simulink model "generic_src"  (Simulink 10.3)
settings: Solver=ode45  StartTime=0.0  StopTime=inf  RelTol=1e-3  EnableMultiTasking=on
undefined symbols (not defined in the file or in its folder): Area_Front, Area_Rear, ay_max_off, ay_max_on, ay_per_mu_max_off, ay_per_mu_max_on, Brake_ratio, brake_valve_ctrl_kP, cat1mode1_higher, cat1mode1_lower, cat1mode2_higher, cat1mode2_lower, cat1mode3_higher, cat1mode3_lower, cat2mode1_higher, cat2mode1_lower, cat2mode2_higher, cat2mode2_lower, cat2mode3_higher, cat2mode3_lower, delta_vel, diff_lock_fac, diff_lock_off, diff_lock_on, ESP_ctrl_kD, ESP_ctrl_kI, ESP_ctrl_kP, ESP_ctrl_restore_kI, ESP_min_throttle_fac, f_ax, f_slip, g, higherlimit_highvel, higherlimit_lowvel, highervel_fac, highervelocity_fac, InitialConditionForIntegrator, limit_acc, limit_selectlow, limit_starting, limit_vdiff, locktime_throttle, lowerlimit_highvel, lowerlimit_lowvel, lowervel_fac, lowervelocity_fac, min_throttle, MPS2KMPH, MSR_ctrl_kD, MSR_ctrl_kI, MSR_ctrl_kP, MSR_min_throttle_fac, PID_kP_sideslip, PID_kP_yawrate, RADpS2RpM, rBrake, RpM2RADpS, SH_SL_switch, sideslip_vel_corr, sidesplip_deviation_max ... (+35)
libraries: CarMaker4SL x137, simulink x57, simulink_extras x6
(part 6 of 12)

== system generic_src/CarMaker/IPG Vehicle/PowerTrain/PTControl Example/PTControl_In/CreateBus PTC GearboxIn5 ==
  In : Inport
  BusCreator : BusCreator  Inputs=20
  Demux : Demux  Outputs=20
      settings: DisplayOption=none
  Out : Outport  VectorParamsAs1DForOutWhenUnconnected=off
  wires:
  Demux/20 -> BusCreator/20  "PTC GearboxIn5 Clutch_dis i_TrqIn2Out"
  Demux/19 -> BusCreator/19  "PTC GearboxIn5 Clutch_dis Trq_out"
  Demux/18 -> BusCreator/18  "PTC GearboxIn5 Clutch_dis Trq_in"
  Demux/17 -> BusCreator/17  "PTC GearboxIn5 Clutch_dis rotv_out"
  Demux/16 -> BusCreator/16  "PTC GearboxIn5 Clutch_dis rotv_in"
  Demux/15 -> BusCreator/15  "PTC GearboxIn5 Clutch_dis Pos"
  Demux/14 -> BusCreator/14  "PTC GearboxIn5 Clutch i_TrqIn2Out"
  Demux/13 -> BusCreator/13  "PTC GearboxIn5 Clutch Trq_out"
  Demux/12 -> BusCreator/12  "PTC GearboxIn5 Clutch Trq_in"
  Demux/11 -> BusCreator/11  "PTC GearboxIn5 Clutch rotv_out"
  Demux/10 -> BusCreator/10  "PTC GearboxIn5 Clutch rotv_in"
  Demux/9 -> BusCreator/9  "PTC GearboxIn5 Clutch Pos"
  Demux/8 -> BusCreator/8  "PTC GearboxIn5 Trq_out"
  Demux/7 -> BusCreator/7  "PTC GearboxIn5 Trq_in"
  Demux/6 -> BusCreator/6  "PTC GearboxIn5 rotv_out"
  Demux/5 -> BusCreator/5  "PTC GearboxIn5 rotv_in"
  Demux/4 -> BusCreator/4  "PTC GearboxIn5 i"
  Demux/3 -> BusCreator/3  "PTC GearboxIn5 Trq_DriveSrc_trg"
  Demux/2 -> BusCreator/2  "PTC GearboxIn5 GearNo_dis"
  Demux/1 -> BusCreator/1  "PTC GearboxIn5 GearNo"
  BusCreator/1 -> Out/1
  In/1 -> Demux/1

== system generic_src/CarMaker/IPG Vehicle/PowerTrain/PTControl Example/PTControl_In/CreateBus PTC GearboxIn6 ==
  In : Inport
  BusCreator : BusCreator  Inputs=20
  Demux : Demux  Outputs=20
      settings: DisplayOption=none
  Out : Outport  VectorParamsAs1DForOutWhenUnconnected=off
  wires:
  Demux/20 -> BusCreator/20  "PTC GearboxIn6 Clutch_dis i_TrqIn2Out"
  Demux/19 -> BusCreator/19  "PTC GearboxIn6 Clutch_dis Trq_out"
  Demux/18 -> BusCreator/18  "PTC GearboxIn6 Clutch_dis Trq_in"
  Demux/17 -> BusCreator/17  "PTC GearboxIn6 Clutch_dis rotv_out"
  Demux/16 -> BusCreator/16  "PTC GearboxIn6 Clutch_dis rotv_in"
  Demux/15 -> BusCreator/15  "PTC GearboxIn6 Clutch_dis Pos"
  Demux/14 -> BusCreator/14  "PTC GearboxIn6 Clutch i_TrqIn2Out"
  Demux/13 -> BusCreator/13  "PTC GearboxIn6 Clutch Trq_out"
  Demux/12 -> BusCreator/12  "PTC GearboxIn6 Clutch Trq_in"
  Demux/11 -> BusCreator/11  "PTC GearboxIn6 Clutch rotv_out"
  Demux/10 -> BusCreator/10  "PTC GearboxIn6 Clutch rotv_in"
  Demux/9 -> BusCreator/9  "PTC GearboxIn6 Clutch Pos"
  Demux/8 -> BusCreator/8  "PTC GearboxIn6 Trq_out"
  Demux/7 -> BusCreator/7  "PTC GearboxIn6 Trq_in"
  Demux/6 -> BusCreator/6  "PTC GearboxIn6 rotv_out"
  Demux/5 -> BusCreator/5  "PTC GearboxIn6 rotv_in"
  Demux/4 -> BusCreator/4  "PTC GearboxIn6 i"
  Demux/3 -> BusCreator/3  "PTC GearboxIn6 Trq_DriveSrc_trg"
  Demux/2 -> BusCreator/2  "PTC GearboxIn6 GearNo_dis"
  Demux/1 -> BusCreator/1  "PTC GearboxIn6 GearNo"
  BusCreator/1 -> Out/1
  In/1 -> Demux/1

== system generic_src/CarMaker/IPG Vehicle/PowerTrain/PTControl Example/PTControl_In/CreateBus PTC GearboxIn7 ==
  In : Inport
  BusCreator : BusCreator  Inputs=20
  Demux : Demux  Outputs=20
      settings: DisplayOption=none
  Out : Outport  VectorParamsAs1DForOutWhenUnconnected=off
  wires:
  Demux/20 -> BusCreator/20  "PTC GearboxIn7 Clutch_dis i_TrqIn2Out"
  Demux/19 -> BusCreator/19  "PTC GearboxIn7 Clutch_dis Trq_out"
  Demux/18 -> BusCreator/18  "PTC GearboxIn7 Clutch_dis Trq_in"
  Demux/17 -> BusCreator/17  "PTC GearboxIn7 Clutch_dis rotv_out"
  Demux/16 -> BusCreator/16  "PTC GearboxIn7 Clutch_dis rotv_in"
  Demux/15 -> BusCreator/15  "PTC GearboxIn7 Clutch_dis Pos"
  Demux/14 -> BusCreator/14  "PTC GearboxIn7 Clutch i_TrqIn2Out"
  Demux/13 -> BusCreator/13  "PTC GearboxIn7 Clutch Trq_out"
  Demux/12 -> BusCreator/12  "PTC GearboxIn7 Clutch Trq_in"
  Demux/11 -> BusCreator/11  "PTC GearboxIn7 Clutch rotv_out"
  Demux/10 -> BusCreator/10  "PTC GearboxIn7 Clutch rotv_in"
  Demux/9 -> BusCreator/9  "PTC GearboxIn7 Clutch Pos"
  Demux/8 -> BusCreator/8  "PTC GearboxIn7 Trq_out"
  Demux/7 -> BusCreator/7  "PTC GearboxIn7 Trq_in"
  Demux/6 -> BusCreator/6  "PTC GearboxIn7 rotv_out"
  Demux/5 -> BusCreator/5  "PTC GearboxIn7 rotv_in"
  Demux/4 -> BusCreator/4  "PTC GearboxIn7 i"
  Demux/3 -> BusCreator/3  "PTC GearboxIn7 Trq_DriveSrc_trg"
  Demux/2 -> BusCreator/2  "PTC GearboxIn7 GearNo_dis"
  Demux/1 -> BusCreator/1  "PTC GearboxIn7 GearNo"
  BusCreator/1 -> Out/1
  In/1 -> Demux/1

== system generic_src/CarMaker/IPG Vehicle/PowerTrain/PTControl Example/PTControl_In/CreateBus PTC GearboxIn8 ==
  In : Inport
  BusCreator : BusCreator  Inputs=20
  Demux : Demux  Outputs=20
      settings: DisplayOption=none
  Out : Outport  VectorParamsAs1DForOutWhenUnconnected=off
  wires:
  Demux/20 -> BusCreator/20  "PTC GearboxIn8 Clutch_dis i_TrqIn2Out"
  Demux/19 -> BusCreator/19  "PTC GearboxIn8 Clutch_dis Trq_out"
  Demux/18 -> BusCreator/18  "PTC GearboxIn8 Clutch_dis Trq_in"
  Demux/17 -> BusCreator/17  "PTC GearboxIn8 Clutch_dis rotv_out"
  Demux/16 -> BusCreator/16  "PTC GearboxIn8 Clutch_dis rotv_in"
  Demux/15 -> BusCreator/15  "PTC GearboxIn8 Clutch_dis Pos"
  Demux/14 -> BusCreator/14  "PTC GearboxIn8 Clutch i_TrqIn2Out"
  Demux/13 -> BusCreator/13  "PTC GearboxIn8 Clutch Trq_out"
  Demux/12 -> BusCreator/12  "PTC GearboxIn8 Clutch Trq_in"
  Demux/11 -> BusCreator/11  "PTC GearboxIn8 Clutch rotv_out"
  Demux/10 -> BusCreator/10  "PTC GearboxIn8 Clutch rotv_in"
  Demux/9 -> BusCreator/9  "PTC GearboxIn8 Clutch Pos"
  Demux/8 -> BusCreator/8  "PTC GearboxIn8 Trq_out"
  Demux/7 -> BusCreator/7  "PTC GearboxIn8 Trq_in"
  Demux/6 -> BusCreator/6  "PTC GearboxIn8 rotv_out"
  Demux/5 -> BusCreator/5  "PTC GearboxIn8 rotv_in"
  Demux/4 -> BusCreator/4  "PTC GearboxIn8 i"
  Demux/3 -> BusCreator/3  "PTC GearboxIn8 Trq_DriveSrc_trg"
  Demux/2 -> BusCreator/2  "PTC GearboxIn8 GearNo_dis"
  Demux/1 -> BusCreator/1  "PTC GearboxIn8 GearNo"
  BusCreator/1 -> Out/1
  In/1 -> Demux/1

== system generic_src/CarMaker/IPG Vehicle/PowerTrain/PTControl Example/PTControl_In/CreateBus PTC GearboxIn9 ==
  In : Inport
  BusCreator : BusCreator  Inputs=20
  Demux : Demux  Outputs=20
      settings: DisplayOption=none
  Out : Outport  VectorParamsAs1DForOutWhenUnconnected=off
  wires:
  Demux/20 -> BusCreator/20  "PTC GearboxIn9 Clutch_dis i_TrqIn2Out"
  Demux/19 -> BusCreator/19  "PTC GearboxIn9 Clutch_dis Trq_out"
  Demux/18 -> BusCreator/18  "PTC GearboxIn9 Clutch_dis Trq_in"
  Demux/17 -> BusCreator/17  "PTC GearboxIn9 Clutch_dis rotv_out"
  Demux/16 -> BusCreator/16  "PTC GearboxIn9 Clutch_dis rotv_in"
  Demux/15 -> BusCreator/15  "PTC GearboxIn9 Clutch_dis Pos"
  Demux/14 -> BusCreator/14  "PTC GearboxIn9 Clutch i_TrqIn2Out"
  Demux/13 -> BusCreator/13  "PTC GearboxIn9 Clutch Trq_out"
  Demux/12 -> BusCreator/12  "PTC GearboxIn9 Clutch Trq_in"
  Demux/11 -> BusCreator/11  "PTC GearboxIn9 Clutch rotv_out"
  Demux/10 -> BusCreator/10  "PTC GearboxIn9 Clutch rotv_in"
  Demux/9 -> BusCreator/9  "PTC GearboxIn9 Clutch Pos"
  Demux/8 -> BusCreator/8  "PTC GearboxIn9 Trq_out"
  Demux/7 -> BusCreator/7  "PTC GearboxIn9 Trq_in"
  Demux/6 -> BusCreator/6  "PTC GearboxIn9 rotv_out"
  Demux/5 -> BusCreator/5  "PTC GearboxIn9 rotv_in"
  Demux/4 -> BusCreator/4  "PTC GearboxIn9 i"
  Demux/3 -> BusCreator/3  "PTC GearboxIn9 Trq_DriveSrc_trg"
  Demux/2 -> BusCreator/2  "PTC GearboxIn9 GearNo_dis"
  Demux/1 -> BusCreator/1  "PTC GearboxIn9 GearNo"
  BusCreator/1 -> Out/1
  In/1 -> Demux/1

== system generic_src/CarMaker/IPG Vehicle/PowerTrain/PTControl Example/PTControl_In/CreateBus PTC ISGIn ==
  In : Inport
  BusCreator : BusCreator  Inputs=9
  Demux : Demux  Outputs=9
      settings: DisplayOption=none
  Out : Outport  VectorParamsAs1DForOutWhenUnconnected=off
  wires:
  Demux/9 -> BusCreator/9  "PTC ISGIn i_M2W_RR"
  Demux/8 -> BusCreator/8  "PTC ISGIn i_M2W_RL"
  Demux/7 -> BusCreator/7  "PTC ISGIn i_M2W_FR"
  Demux/6 -> BusCreator/6  "PTC ISGIn i_M2W_FL"
  Demux/5 -> BusCreator/5  "PTC ISGIn PwrElec"
  Demux/4 -> BusCreator/4  "PTC ISGIn TrqGen_max"
  Demux/3 -> BusCreator/3  "PTC ISGIn TrqMot_max"
  Demux/2 -> BusCreator/2  "PTC ISGIn Trq"
  Demux/1 -> BusCreator/1  "PTC ISGIn rotv"
  BusCreator/1 -> Out/1
  In/1 -> Demux/1

== system generic_src/CarMaker/IPG Vehicle/PowerTrain/PTControl Example/PTControl_In/CreateBus PTC MotorIn0 ==
  In : Inport
  BusCreator : BusCreator  Inputs=9
  Demux : Demux  Outputs=9
      settings: DisplayOption=none
  Out : Outport  VectorParamsAs1DForOutWhenUnconnected=off
  wires:
  Demux/9 -> BusCreator/9  "PTC MotorIn0 i_M2W_RR"
  Demux/8 -> BusCreator/8  "PTC MotorIn0 i_M2W_RL"
  Demux/7 -> BusCreator/7  "PTC MotorIn0 i_M2W_FR"
  Demux/6 -> BusCreator/6  "PTC MotorIn0 i_M2W_FL"
  Demux/5 -> BusCreator/5  "PTC MotorIn0 PwrElec"
  Demux/4 -> BusCreator/4  "PTC MotorIn0 TrqGen_max"
  Demux/3 -> BusCreator/3  "PTC MotorIn0 TrqMot_max"
  Demux/2 -> BusCreator/2  "PTC MotorIn0 Trq"
  Demux/1 -> BusCreator/1  "PTC MotorIn0 rotv"
  BusCreator/1 -> Out/1
  In/1 -> Demux/1

== system generic_src/CarMaker/IPG Vehicle/PowerTrain/PTControl Example/PTControl_In/CreateBus PTC MotorIn1 ==
  In : Inport
  BusCreator : BusCreator  Inputs=9
  Demux : Demux  Outputs=9
      settings: DisplayOption=none
  Out : Outport  VectorParamsAs1DForOutWhenUnconnected=off
  wires:
  Demux/9 -> BusCreator/9  "PTC MotorIn1 i_M2W_RR"
  Demux/8 -> BusCreator/8  "PTC MotorIn1 i_M2W_RL"
  Demux/7 -> BusCreator/7  "PTC MotorIn1 i_M2W_FR"
  Demux/6 -> BusCreator/6  "PTC MotorIn1 i_M2W_FL"
  Demux/5 -> BusCreator/5  "PTC MotorIn1 PwrElec"
  Demux/4 -> BusCreator/4  "PTC MotorIn1 TrqGen_max"
  Demux/3 -> BusCreator/3  "PTC MotorIn1 TrqMot_max"
  Demux/2 -> BusCreator/2  "PTC MotorIn1 Trq"
  Demux/1 -> BusCreator/1  "PTC MotorIn1 rotv"
  BusCreator/1 -> Out/1
  In/1 -> Demux/1

== system generic_src/CarMaker/IPG Vehicle/PowerTrain/PTControl Example/PTControl_In/CreateBus PTC MotorIn10 ==
  In : Inport
  BusCreator : BusCreator  Inputs=9
  Demux : Demux  Outputs=9
      settings: DisplayOption=none
  Out : Outport  VectorParamsAs1DForOutWhenUnconnected=off
  wires:
  Demux/9 -> BusCreator/9  "PTC MotorIn10 i_M2W_RR"
  Demux/8 -> BusCreator/8  "PTC MotorIn10 i_M2W_RL"
  Demux/7 -> BusCreator/7  "PTC MotorIn10 i_M2W_FR"
  Demux/6 -> BusCreator/6  "PTC MotorIn10 i_M2W_FL"
  Demux/5 -> BusCreator/5  "PTC MotorIn10 PwrElec"
  Demux/4 -> BusCreator/4  "PTC MotorIn10 TrqGen_max"
  Demux/3 -> BusCreator/3  "PTC MotorIn10 TrqMot_max"
  Demux/2 -> BusCreator/2  "PTC MotorIn10 Trq"
  Demux/1 -> BusCreator/1  "PTC MotorIn10 rotv"
  BusCreator/1 -> Out/1
  In/1 -> Demux/1

== system generic_src/CarMaker/IPG Vehicle/PowerTrain/PTControl Example/PTControl_In/CreateBus PTC MotorIn11 ==
  In : Inport
  BusCreator : BusCreator  Inputs=9
  Demux : Demux  Outputs=9
      settings: DisplayOption=none
  Out : Outport  VectorParamsAs1DForOutWhenUnconnected=off
  wires:
  Demux/9 -> BusCreator/9  "PTC MotorIn11 i_M2W_RR"
  Demux/8 -> BusCreator/8  "PTC MotorIn11 i_M2W_RL"
  Demux/7 -> BusCreator/7  "PTC MotorIn11 i_M2W_FR"
  Demux/6 -> BusCreator/6  "PTC MotorIn11 i_M2W_FL"
  Demux/5 -> BusCreator/5  "PTC MotorIn11 PwrElec"
  Demux/4 -> BusCreator/4  "PTC MotorIn11 TrqGen_max"
  Demux/3 -> BusCreator/3  "PTC MotorIn11 TrqMot_max"
  Demux/2 -> BusCreator/2  "PTC MotorIn11 Trq"
  Demux/1 -> BusCreator/1  "PTC MotorIn11 rotv"
  BusCreator/1 -> Out/1
  In/1 -> Demux/1

== system generic_src/CarMaker/IPG Vehicle/PowerTrain/PTControl Example/PTControl_In/CreateBus PTC MotorIn2 ==
  In : Inport
  BusCreator : BusCreator  Inputs=9
  Demux : Demux  Outputs=9
      settings: DisplayOption=none
  Out : Outport  VectorParamsAs1DForOutWhenUnconnected=off
  wires:
  Demux/9 -> BusCreator/9  "PTC MotorIn2 i_M2W_RR"
  Demux/8 -> BusCreator/8  "PTC MotorIn2 i_M2W_RL"
  Demux/7 -> BusCreator/7  "PTC MotorIn2 i_M2W_FR"
  Demux/6 -> BusCreator/6  "PTC MotorIn2 i_M2W_FL"
  Demux/5 -> BusCreator/5  "PTC MotorIn2 PwrElec"
  Demux/4 -> BusCreator/4  "PTC MotorIn2 TrqGen_max"
  Demux/3 -> BusCreator/3  "PTC MotorIn2 TrqMot_max"
  Demux/2 -> BusCreator/2  "PTC MotorIn2 Trq"
  Demux/1 -> BusCreator/1  "PTC MotorIn2 rotv"
  BusCreator/1 -> Out/1
  In/1 -> Demux/1

== system generic_src/CarMaker/IPG Vehicle/PowerTrain/PTControl Example/PTControl_In/CreateBus PTC MotorIn3 ==
  In : Inport
  BusCreator : BusCreator  Inputs=9
  Demux : Demux  Outputs=9
      settings: DisplayOption=none
  Out : Outport  VectorParamsAs1DForOutWhenUnconnected=off
  wires:
  Demux/9 -> BusCreator/9  "PTC MotorIn3 i_M2W_RR"
  Demux/8 -> BusCreator/8  "PTC MotorIn3 i_M2W_RL"
  Demux/7 -> BusCreator/7  "PTC MotorIn3 i_M2W_FR"
  Demux/6 -> BusCreator/6  "PTC MotorIn3 i_M2W_FL"
  Demux/5 -> BusCreator/5  "PTC MotorIn3 PwrElec"
  Demux/4 -> BusCreator/4  "PTC MotorIn3 TrqGen_max"
  Demux/3 -> BusCreator/3  "PTC MotorIn3 TrqMot_max"
  Demux/2 -> BusCreator/2  "PTC MotorIn3 Trq"
  Demux/1 -> BusCreator/1  "PTC MotorIn3 rotv"
  BusCreator/1 -> Out/1
  In/1 -> Demux/1

== system generic_src/CarMaker/IPG Vehicle/PowerTrain/PTControl Example/PTControl_In/CreateBus PTC MotorIn4 ==
  In : Inport
  BusCreator : BusCreator  Inputs=9
  Demux : Demux  Outputs=9
      settings: DisplayOption=none
  Out : Outport  VectorParamsAs1DForOutWhenUnconnected=off
  wires:
  Demux/9 -> BusCreator/9  "PTC MotorIn4 i_M2W_RR"
  Demux/8 -> BusCreator/8  "PTC MotorIn4 i_M2W_RL"
  Demux/7 -> BusCreator/7  "PTC MotorIn4 i_M2W_FR"
  Demux/6 -> BusCreator/6  "PTC MotorIn4 i_M2W_FL"
  Demux/5 -> BusCreator/5  "PTC MotorIn4 PwrElec"
  Demux/4 -> BusCreator/4  "PTC MotorIn4 TrqGen_max"
  Demux/3 -> BusCreator/3  "PTC MotorIn4 TrqMot_max"
  Demux/2 -> BusCreator/2  "PTC MotorIn4 Trq"
  Demux/1 -> BusCreator/1  "PTC MotorIn4 rotv"
  BusCreator/1 -> Out/1
  In/1 -> Demux/1

== system generic_src/CarMaker/IPG Vehicle/PowerTrain/PTControl Example/PTControl_In/CreateBus PTC MotorIn5 ==
  In : Inport
  BusCreator : BusCreator  Inputs=9
  Demux : Demux  Outputs=9
      settings: DisplayOption=none
  Out : Outport  VectorParamsAs1DForOutWhenUnconnected=off
  wires:
  Demux/9 -> BusCreator/9  "PTC MotorIn5 i_M2W_RR"
  Demux/8 -> BusCreator/8  "PTC MotorIn5 i_M2W_RL"
  Demux/7 -> BusCreator/7  "PTC MotorIn5 i_M2W_FR"
  Demux/6 -> BusCreator/6  "PTC MotorIn5 i_M2W_FL"
  Demux/5 -> BusCreator/5  "PTC MotorIn5 PwrElec"
  Demux/4 -> BusCreator/4  "PTC MotorIn5 TrqGen_max"
  Demux/3 -> BusCreator/3  "PTC MotorIn5 TrqMot_max"
  Demux/2 -> BusCreator/2  "PTC MotorIn5 Trq"
  Demux/1 -> BusCreator/1  "PTC MotorIn5 rotv"
  BusCreator/1 -> Out/1
  In/1 -> Demux/1

== system generic_src/CarMaker/IPG Vehicle/PowerTrain/PTControl Example/PTControl_In/CreateBus PTC MotorIn6 ==
  In : Inport
  BusCreator : BusCreator  Inputs=9
  Demux : Demux  Outputs=9
      settings: DisplayOption=none
  Out : Outport  VectorParamsAs1DForOutWhenUnconnected=off
  wires:
  Demux/9 -> BusCreator/9  "PTC MotorIn6 i_M2W_RR"
  Demux/8 -> BusCreator/8  "PTC MotorIn6 i_M2W_RL"
  Demux/7 -> BusCreator/7  "PTC MotorIn6 i_M2W_FR"
  Demux/6 -> BusCreator/6  "PTC MotorIn6 i_M2W_FL"
  Demux/5 -> BusCreator/5  "PTC MotorIn6 PwrElec"
  Demux/4 -> BusCreator/4  "PTC MotorIn6 TrqGen_max"
  Demux/3 -> BusCreator/3  "PTC MotorIn6 TrqMot_max"
  Demux/2 -> BusCreator/2  "PTC MotorIn6 Trq"
  Demux/1 -> BusCreator/1  "PTC MotorIn6 rotv"
  BusCreator/1 -> Out/1
  In/1 -> Demux/1

== system generic_src/CarMaker/IPG Vehicle/PowerTrain/PTControl Example/PTControl_In/CreateBus PTC MotorIn7 ==
  In : Inport
  BusCreator : BusCreator  Inputs=9
  Demux : Demux  Outputs=9
      settings: DisplayOption=none
  Out : Outport  VectorParamsAs1DForOutWhenUnconnected=off
  wires:
  Demux/9 -> BusCreator/9  "PTC MotorIn7 i_M2W_RR"
  Demux/8 -> BusCreator/8  "PTC MotorIn7 i_M2W_RL"
  Demux/7 -> BusCreator/7  "PTC MotorIn7 i_M2W_FR"
  Demux/6 -> BusCreator/6  "PTC MotorIn7 i_M2W_FL"
  Demux/5 -> BusCreator/5  "PTC MotorIn7 PwrElec"
  Demux/4 -> BusCreator/4  "PTC MotorIn7 TrqGen_max"
  Demux/3 -> BusCreator/3  "PTC MotorIn7 TrqMot_max"
  Demux/2 -> BusCreator/2  "PTC MotorIn7 Trq"
  Demux/1 -> BusCreator/1  "PTC MotorIn7 rotv"
  BusCreator/1 -> Out/1
  In/1 -> Demux/1

== system generic_src/CarMaker/IPG Vehicle/PowerTrain/PTControl Example/PTControl_In/CreateBus PTC MotorIn8 ==
  In : Inport
  BusCreator : BusCreator  Inputs=9
  Demux : Demux  Outputs=9
      settings: DisplayOption=none
  Out : Outport  VectorParamsAs1DForOutWhenUnconnected=off
  wires:
  Demux/9 -> BusCreator/9  "PTC MotorIn8 i_M2W_RR"
  Demux/8 -> BusCreator/8  "PTC MotorIn8 i_M2W_RL"
  Demux/7 -> BusCreator/7  "PTC MotorIn8 i_M2W_FR"
  Demux/6 -> BusCreator/6  "PTC MotorIn8 i_M2W_FL"
  Demux/5 -> BusCreator/5  "PTC MotorIn8 PwrElec"
  Demux/4 -> BusCreator/4  "PTC MotorIn8 TrqGen_max"
  Demux/3 -> BusCreator/3  "PTC MotorIn8 TrqMot_max"
  Demux/2 -> BusCreator/2  "PTC MotorIn8 Trq"
  Demux/1 -> BusCreator/1  "PTC MotorIn8 rotv"
  BusCreator/1 -> Out/1
  In/1 -> Demux/1

== system generic_src/CarMaker/IPG Vehicle/PowerTrain/PTControl Example/PTControl_In/CreateBus PTC MotorIn9 ==
  In : Inport
  BusCreator : BusCreator  Inputs=9
  Demux : Demux  Outputs=9
      settings: DisplayOption=none
  Out : Outport  VectorParamsAs1DForOutWhenUnconnected=off
  wires:
  Demux/9 -> BusCreator/9  "PTC MotorIn9 i_M2W_RR"
  Demux/8 -> BusCreator/8  "PTC MotorIn9 i_M2W_RL"
  Demux/7 -> BusCreator/7  "PTC MotorIn9 i_M2W_FR"
  Demux/6 -> BusCreator/6  "PTC MotorIn9 i_M2W_FL"
  Demux/5 -> BusCreator/5  "PTC MotorIn9 PwrElec"
  Demux/4 -> BusCreator/4  "PTC MotorIn9 TrqGen_max"
  Demux/3 -> BusCreator/3  "PTC MotorIn9 TrqMot_max"
  Demux/2 -> BusCreator/2  "PTC MotorIn9 Trq"
  Demux/1 -> BusCreator/1  "PTC MotorIn9 rotv"
  BusCreator/1 -> Out/1
  In/1 -> Demux/1

== system generic_src/CarMaker/IPG Vehicle/PowerTrain/PTControl Example/PTControl_In/CreateBus PTC PwrSupplyIn ==
  In : Inport
  BusCreator : BusCreator  Inputs=12
  Demux : Demux  Outputs=12
      settings: DisplayOption=none
  Out : Outport  VectorParamsAs1DForOutWhenUnconnected=off
  wires:
  Demux/12 -> BusCreator/12  "PTC PwrSupplyIn Eta_HV1toHV2"
  Demux/11 -> BusCreator/11  "PTC PwrSupplyIn Eta_HV1toLV"
  Demux/10 -> BusCreator/10  "PTC PwrSupplyIn Pwr_HV1toHV2_max"
  Demux/9 -> BusCreator/9  "PTC PwrSupplyIn Pwr_HV1toLV_max"
  Demux/8 -> BusCreator/8  "PTC PwrSupplyIn Pwr_HV1toHV2"
  Demux/7 -> BusCreator/7  "PTC PwrSupplyIn Pwr_HV1toLV"
  Demux/6 -> BusCreator/6  "PTC PwrSupplyIn Voltage_HV2"
  Demux/5 -> BusCreator/5  "PTC PwrSupplyIn Voltage_HV1"
  Demux/4 -> BusCreator/4  "PTC PwrSupplyIn Voltage_LV"
  Demux/3 -> BusCreator/3  "PTC PwrSupplyIn Pwr_HV2"
  Demux/2 -> BusCreator/2  "PTC PwrSupplyIn Pwr_HV1"
  Demux/1 -> BusCreator/1  "PTC PwrSupplyIn Pwr_LV"
  BusCreator/1 -> Out/1
  In/1 -> Demux/1

== system generic_src/CarMaker/IPG Vehicle/PowerTrain/PTControl Example/PTControl_In/CreateBus PTC Vehicle Ctrl ==
  In : Inport
  BusCreator : BusCreator  Inputs=8
  Demux : Demux  Outputs=8
      settings: DisplayOption=none
  Out : Outport  VectorParamsAs1DForOutWhenUnconnected=off
  wires:
  Demux/8 -> BusCreator/8  "PTC Velocity"
  Demux/7 -> BusCreator/7  "PTC Brake"
  Demux/6 -> BusCreator/6  "PTC Gas"
  Demux/5 -> BusCreator/5  "PTC Clutch"
  Demux/4 -> BusCreator/4  "PTC GearNoTrg"
  Demux/3 -> BusCreator/3  "PTC SelectorCtrl"
  Demux/2 -> BusCreator/2  "PTC SST"
  Demux/1 -> BusCreator/1  "PTC Key"
  BusCreator/1 -> Out/1
  In/1 -> Demux/1

== system generic_src/CarMaker/IPG Vehicle/PowerTrain/PTControl Example/PTControl_In/CreateBus PTC WheelIn ==
  In : Inport
  BusCreator : BusCreator  Inputs=4
  Demux : Demux
      settings: DisplayOption=none
  Out : Outport  VectorParamsAs1DForOutWhenUnconnected=off
  wires:
  Demux/4 -> BusCreator/4  "PTC WheelIn_RR Trq_BrakeReg_trg"
  Demux/3 -> BusCreator/3  "PTC WheelIn_RL Trq_BrakeReg_trg"
  Demux/2 -> BusCreator/2  "PTC WheelIn_FR Trq_BrakeReg_trg"
  Demux/1 -> BusCreator/1  "PTC WheelIn_FL Trq_BrakeReg_trg"
  BusCreator/1 -> Out/1
  In/1 -> Demux/1

== system generic_src/CarMaker/IPG Vehicle/PowerTrain/PTControl Example/PTControl_In/CreateBus PTC_Cfg BatteryHV ==
  In : Inport
  BusCreator : BusCreator  Inputs=6
  Demux : Demux  Outputs=6
      settings: DisplayOption=none
  Out : Outport  VectorParamsAs1DForOutWhenUnconnected=off
  wires:
  Demux/2 -> BusCreator/2  "PTC_Cfg BattHV SOC_max"
  Demux/5 -> BusCreator/5  "PTC_Cfg BattHV Temp_init"
  Demux/6 -> BusCreator/6  "PTC_Cfg BattHV TempCool_init"
  Demux/1 -> BusCreator/1  "PTC_Cfg BattHV SOC_min"
  BusCreator/1 -> Out/1
  Demux/4 -> BusCreator/4  "PTC_Cfg BattHV Voltage"
  In/1 -> Demux/1
  Demux/3 -> BusCreator/3  "PTC_Cfg BattHV Capacity"

== system generic_src/CarMaker/IPG Vehicle/PowerTrain/PTControl Example/PTControl_In/CreateBus PTC_Cfg BatteryLV ==
  In : Inport
  BusCreator : BusCreator  Inputs=6
  Demux : Demux  Outputs=6
      settings: DisplayOption=none
  Out : Outport  VectorParamsAs1DForOutWhenUnconnected=off
  wires:
  Demux/3 -> BusCreator/3  "PTC_Cfg BattLV Capacity"
  In/1 -> Demux/1
  Demux/4 -> BusCreator/4  "PTC_Cfg BattLV Voltage"
  BusCreator/1 -> Out/1
  Demux/1 -> BusCreator/1  "PTC_Cfg BattLV SOC_min"
  Demux/6 -> BusCreator/6  "PTC_Cfg BattLV TempCool_init"
  Demux/5 -> BusCreator/5  "PTC_Cfg BattLV Temp_init"
  Demux/2 -> BusCreator/2  "PTC_Cfg BattLV SOC_max"

== system generic_src/CarMaker/IPG Vehicle/PowerTrain/PTControl Example/PTControl_In/CreateBus PTC_Cfg Engine ==
  In : Inport
  BusCreator : BusCreator  Inputs=4
  Demux : Demux
      settings: DisplayOption=none
  Out : Outport  VectorParamsAs1DForOutWhenUnconnected=off
  wires:
  Demux/4 -> BusCreator/4  "PTC_Cfg Engine rotv_opt"
  Demux/3 -> BusCreator/3  "PTC_Cfg Engine rotv_idle"
  Demux/2 -> BusCreator/2  "PTC_Cfg Engine rotv_max"
  Demux/1 -> BusCreator/1  "PTC_Cfg Engine Fuel_l2kWh"
  BusCreator/1 -> Out/1
  In/1 -> Demux/1

== system generic_src/CarMaker/IPG Vehicle/PowerTrain/PTControl Example/PTControl_In/CreateBus PTC_Cfg GearBox0 ==
  In : Inport
  BusCreator : BusCreator  Inputs=38
  Demux : Demux  Outputs=38
      settings: DisplayOption=none
  Out : Outport  VectorParamsAs1DForOutWhenUnconnected=off
  wires:
  Demux/38 -> BusCreator/38  "PTC_Cfg GearBox0 iBGear16"
  Demux/37 -> BusCreator/37  "PTC_Cfg GearBox0 iBGear15"
  Demux/36 -> BusCreator/36  "PTC_Cfg GearBox0 iBGear14"
  Demux/35 -> BusCreator/35  "PTC_Cfg GearBox0 iBGear13"
  Demux/34 -> BusCreator/34  "PTC_Cfg GearBox0 iBGear12"
  Demux/33 -> BusCreator/33  "PTC_Cfg GearBox0 iBGear11"
  Demux/32 -> BusCreator/32  "PTC_Cfg GearBox0 iBGear10"
  Demux/31 -> BusCreator/31  "PTC_Cfg GearBox0 iBGear9"
  Demux/30 -> BusCreator/30  "PTC_Cfg GearBox0 iBGear8"
  Demux/29 -> BusCreator/29  "PTC_Cfg GearBox0 iBGear7"
  Demux/28 -> BusCreator/28  "PTC_Cfg GearBox0 iBGear6"
  Demux/27 -> BusCreator/27  "PTC_Cfg GearBox0 iBGear5"
  Demux/26 -> BusCreator/26  "PTC_Cfg GearBox0 iBGear4"
  Demux/25 -> BusCreator/25  "PTC_Cfg GearBox0 iBGear3"
  Demux/24 -> BusCreator/24  "PTC_Cfg GearBox0 iBGear2"
  Demux/23 -> BusCreator/23  "PTC_Cfg GearBox0 iBGear1"
  Demux/22 -> BusCreator/22  "PTC_Cfg GearBox0 iBGear0"
  Demux/21 -> BusCreator/21  "PTC_Cfg GearBox0 nBGears"
  Demux/20 -> BusCreator/20  "PTC_Cfg GearBox0 iFGear16"
  Demux/19 -> BusCreator/19  "PTC_Cfg GearBox0 iFGear15"
  Demux/18 -> BusCreator/18  "PTC_Cfg GearBox0 iFGear14"
  Demux/17 -> BusCreator/17  "PTC_Cfg GearBox0 iFGear13"
  Demux/16 -> BusCreator/16  "PTC_Cfg GearBox0 iFGear12"
  Demux/15 -> BusCreator/15  "PTC_Cfg GearBox0 iFGear11"
  Demux/14 -> BusCreator/14  "PTC_Cfg GearBox0 iFGear10"
  Demux/13 -> BusCreator/13  "PTC_Cfg GearBox0 iFGear9"
  Demux/12 -> BusCreator/12  "PTC_Cfg GearBox0 iFGear8"
  Demux/11 -> BusCreator/11  "PTC_Cfg GearBox0 iFGear7"
  Demux/10 -> BusCreator/10  "PTC_Cfg GearBox0 iFGear6"
  Demux/9 -> BusCreator/9  "PTC_Cfg GearBox0 iFGear5"
  Demux/8 -> BusCreator/8  "PTC_Cfg GearBox0 iFGear4"
  Demux/7 -> BusCreator/7  "PTC_Cfg GearBox0 iFGear3"
  Demux/6 -> BusCreator/6  "PTC_Cfg GearBox0 iFGear2"
  Demux/5 -> BusCreator/5  "PTC_Cfg GearBox0 iFGear1"
  Demux/4 -> BusCreator/4  "PTC_Cfg GearBox0 iFGear0"
  Demux/3 -> BusCreator/3  "PTC_Cfg GearBox0 nFGears"
  Demux/2 -> BusCreator/2  "PTC_Cfg GearBox0 ClKind"
  Demux/1 -> BusCreator/1  "PTC_Cfg GearBox0 GBKind"
  BusCreator/1 -> Out/1
  In/1 -> Demux/1

== system generic_src/CarMaker/IPG Vehicle/PowerTrain/PTControl Example/PTControl_In/CreateBus PTC_Cfg GearBox1 ==
  In : Inport
  BusCreator : BusCreator  Inputs=38
  Demux : Demux  Outputs=38
      settings: DisplayOption=none
  Out : Outport  VectorParamsAs1DForOutWhenUnconnected=off
  wires:
  Demux/38 -> BusCreator/38  "PTC_Cfg GearBox1 iBGear16"
  Demux/37 -> BusCreator/37  "PTC_Cfg GearBox1 iBGear15"
  Demux/36 -> BusCreator/36  "PTC_Cfg GearBox1 iBGear14"
  Demux/35 -> BusCreator/35  "PTC_Cfg GearBox1 iBGear13"
  Demux/34 -> BusCreator/34  "PTC_Cfg GearBox1 iBGear12"
  Demux/33 -> BusCreator/33  "PTC_Cfg GearBox1 iBGear11"
  Demux/32 -> BusCreator/32  "PTC_Cfg GearBox1 iBGear10"
  Demux/31 -> BusCreator/31  "PTC_Cfg GearBox1 iBGear9"
  Demux/30 -> BusCreator/30  "PTC_Cfg GearBox1 iBGear8"
  Demux/29 -> BusCreator/29  "PTC_Cfg GearBox1 iBGear7"
  Demux/28 -> BusCreator/28  "PTC_Cfg GearBox1 iBGear6"
  Demux/27 -> BusCreator/27  "PTC_Cfg GearBox1 iBGear5"
  Demux/26 -> BusCreator/26  "PTC_Cfg GearBox1 iBGear4"
  Demux/25 -> BusCreator/25  "PTC_Cfg GearBox1 iBGear3"
  Demux/24 -> BusCreator/24  "PTC_Cfg GearBox1 iBGear2"
  Demux/23 -> BusCreator/23  "PTC_Cfg GearBox1 iBGear1"
  Demux/22 -> BusCreator/22  "PTC_Cfg GearBox1 iBGear0"
  Demux/21 -> BusCreator/21  "PTC_Cfg GearBox1 nBGears"
  Demux/20 -> BusCreator/20  "PTC_Cfg GearBox1 iFGear16"
  Demux/19 -> BusCreator/19  "PTC_Cfg GearBox1 iFGear15"
  Demux/18 -> BusCreator/18  "PTC_Cfg GearBox1 iFGear14"
  Demux/17 -> BusCreator/17  "PTC_Cfg GearBox1 iFGear13"
  Demux/16 -> BusCreator/16  "PTC_Cfg GearBox1 iFGear12"
  Demux/15 -> BusCreator/15  "PTC_Cfg GearBox1 iFGear11"
  Demux/14 -> BusCreator/14  "PTC_Cfg GearBox1 iFGear10"
  Demux/13 -> BusCreator/13  "PTC_Cfg GearBox1 iFGear9"
  Demux/12 -> BusCreator/12  "PTC_Cfg GearBox1 iFGear8"
  Demux/11 -> BusCreator/11  "PTC_Cfg GearBox1 iFGear7"
  Demux/10 -> BusCreator/10  "PTC_Cfg GearBox1 iFGear6"
  Demux/9 -> BusCreator/9  "PTC_Cfg GearBox1 iFGear5"
  Demux/8 -> BusCreator/8  "PTC_Cfg GearBox1 iFGear4"
  Demux/7 -> BusCreator/7  "PTC_Cfg GearBox1 iFGear3"
  Demux/6 -> BusCreator/6  "PTC_Cfg GearBox1 iFGear2"
  Demux/5 -> BusCreator/5  "PTC_Cfg GearBox1 iFGear1"
  Demux/4 -> BusCreator/4  "PTC_Cfg GearBox1 iFGear0"
  Demux/3 -> BusCreator/3  "PTC_Cfg GearBox1 nFGears"
  Demux/2 -> BusCreator/2  "PTC_Cfg GearBox1 ClKind"
  Demux/1 -> BusCreator/1  "PTC_Cfg GearBox1 GBKind"
  BusCreator/1 -> Out/1
  In/1 -> Demux/1

== system generic_src/CarMaker/IPG Vehicle/PowerTrain/PTControl Example/PTControl_In/CreateBus PTC_Cfg Gearbox10 ==
  In : Inport
  BusCreator : BusCreator  Inputs=38
  Demux : Demux  Outputs=38
      settings: DisplayOption=none
  Out : Outport  VectorParamsAs1DForOutWhenUnconnected=off
  wires:
  Demux/38 -> BusCreator/38  "PTC_Cfg Gearbox10 iBGear16"
  Demux/37 -> BusCreator/37  "PTC_Cfg Gearbox10 iBGear15"
  Demux/36 -> BusCreator/36  "PTC_Cfg Gearbox10 iBGear14"
  Demux/35 -> BusCreator/35  "PTC_Cfg Gearbox10 iBGear13"
  Demux/34 -> BusCreator/34  "PTC_Cfg Gearbox10 iBGear12"
  Demux/33 -> BusCreator/33  "PTC_Cfg Gearbox10 iBGear11"
  Demux/32 -> BusCreator/32  "PTC_Cfg Gearbox10 iBGear10"
  Demux/31 -> BusCreator/31  "PTC_Cfg Gearbox10 iBGear9"
  Demux/30 -> BusCreator/30  "PTC_Cfg Gearbox10 iBGear8"
  Demux/29 -> BusCreator/29  "PTC_Cfg Gearbox10 iBGear7"
  Demux/28 -> BusCreator/28  "PTC_Cfg Gearbox10 iBGear6"
  Demux/27 -> BusCreator/27  "PTC_Cfg Gearbox10 iBGear5"
  Demux/26 -> BusCreator/26  "PTC_Cfg Gearbox10 iBGear4"
  Demux/25 -> BusCreator/25  "PTC_Cfg Gearbox10 iBGear3"
  Demux/24 -> BusCreator/24  "PTC_Cfg Gearbox10 iBGear2"
  Demux/23 -> BusCreator/23  "PTC_Cfg Gearbox10 iBGear1"
  Demux/22 -> BusCreator/22  "PTC_Cfg Gearbox10 iBGear0"
  Demux/21 -> BusCreator/21  "PTC_Cfg Gearbox10 nBGears"
  Demux/20 -> BusCreator/20  "PTC_Cfg Gearbox10 iFGear16"
  Demux/19 -> BusCreator/19  "PTC_Cfg Gearbox10 iFGear15"
  Demux/18 -> BusCreator/18  "PTC_Cfg Gearbox10 iFGear14"
  Demux/17 -> BusCreator/17  "PTC_Cfg Gearbox10 iFGear13"
  Demux/16 -> BusCreator/16  "PTC_Cfg Gearbox10 iFGear12"
  Demux/15 -> BusCreator/15  "PTC_Cfg Gearbox10 iFGear11"
  Demux/14 -> BusCreator/14  "PTC_Cfg Gearbox10 iFGear10"
  Demux/13 -> BusCreator/13  "PTC_Cfg Gearbox10 iFGear9"
  Demux/12 -> BusCreator/12  "PTC_Cfg Gearbox10 iFGear8"
  Demux/11 -> BusCreator/11  "PTC_Cfg Gearbox10 iFGear7"
  Demux/10 -> BusCreator/10  "PTC_Cfg Gearbox10 iFGear6"
  Demux/9 -> BusCreator/9  "PTC_Cfg Gearbox10 iFGear5"
  Demux/8 -> BusCreator/8  "PTC_Cfg Gearbox10 iFGear4"
  Demux/7 -> BusCreator/7  "PTC_Cfg Gearbox10 iFGear3"
  Demux/6 -> BusCreator/6  "PTC_Cfg Gearbox10 iFGear2"
  Demux/5 -> BusCreator/5  "PTC_Cfg Gearbox10 iFGear1"
  Demux/4 -> BusCreator/4  "PTC_Cfg Gearbox10 iFGear0"
  Demux/3 -> BusCreator/3  "PTC_Cfg Gearbox10 nFGears"
  Demux/2 -> BusCreator/2  "PTC_Cfg Gearbox10 ClKind"
  Demux/1 -> BusCreator/1  "PTC_Cfg Gearbox10 GBKind"
  BusCreator/1 -> Out/1
  In/1 -> Demux/1

== system generic_src/CarMaker/IPG Vehicle/PowerTrain/PTControl Example/PTControl_In/CreateBus PTC_Cfg Gearbox11 ==
  In : Inport
  BusCreator : BusCreator  Inputs=38
  Demux : Demux  Outputs=38
      settings: DisplayOption=none
  Out : Outport  VectorParamsAs1DForOutWhenUnconnected=off
  wires:
  Demux/38 -> BusCreator/38  "PTC_Cfg Gearbox11 iBGear16"
  Demux/37 -> BusCreator/37  "PTC_Cfg Gearbox11 iBGear15"
  Demux/36 -> BusCreator/36  "PTC_Cfg Gearbox11 iBGear14"
  Demux/35 -> BusCreator/35  "PTC_Cfg Gearbox11 iBGear13"
  Demux/34 -> BusCreator/34  "PTC_Cfg Gearbox11 iBGear12"
  Demux/33 -> BusCreator/33  "PTC_Cfg Gearbox11 iBGear11"
  Demux/32 -> BusCreator/32  "PTC_Cfg Gearbox11 iBGear10"
  Demux/31 -> BusCreator/31  "PTC_Cfg Gearbox11 iBGear9"
  Demux/30 -> BusCreator/30  "PTC_Cfg Gearbox11 iBGear8"
  Demux/29 -> BusCreator/29  "PTC_Cfg Gearbox11 iBGear7"
  Demux/28 -> BusCreator/28  "PTC_Cfg Gearbox11 iBGear6"
  Demux/27 -> BusCreator/27  "PTC_Cfg Gearbox11 iBGear5"
  Demux/26 -> BusCreator/26  "PTC_Cfg Gearbox11 iBGear4"
  Demux/25 -> BusCreator/25  "PTC_Cfg Gearbox11 iBGear3"
  Demux/24 -> BusCreator/24  "PTC_Cfg Gearbox11 iBGear2"
  Demux/23 -> BusCreator/23  "PTC_Cfg Gearbox11 iBGear1"
  Demux/22 -> BusCreator/22  "PTC_Cfg Gearbox11 iBGear0"
  Demux/21 -> BusCreator/21  "PTC_Cfg Gearbox11 nBGears"
  Demux/20 -> BusCreator/20  "PTC_Cfg Gearbox11 iFGear16"
  Demux/19 -> BusCreator/19  "PTC_Cfg Gearbox11 iFGear15"
  Demux/18 -> BusCreator/18  "PTC_Cfg Gearbox11 iFGear14"
  Demux/17 -> BusCreator/17  "PTC_Cfg Gearbox11 iFGear13"
  Demux/16 -> BusCreator/16  "PTC_Cfg Gearbox11 iFGear12"
  Demux/15 -> BusCreator/15  "PTC_Cfg Gearbox11 iFGear11"
  Demux/14 -> BusCreator/14  "PTC_Cfg Gearbox11 iFGear10"
  Demux/13 -> BusCreator/13  "PTC_Cfg Gearbox11 iFGear9"
  Demux/12 -> BusCreator/12  "PTC_Cfg Gearbox11 iFGear8"
  Demux/11 -> BusCreator/11  "PTC_Cfg Gearbox11 iFGear7"
  Demux/10 -> BusCreator/10  "PTC_Cfg Gearbox11 iFGear6"
  Demux/9 -> BusCreator/9  "PTC_Cfg Gearbox11 iFGear5"
  Demux/8 -> BusCreator/8  "PTC_Cfg Gearbox11 iFGear4"
  Demux/7 -> BusCreator/7  "PTC_Cfg Gearbox11 iFGear3"
  Demux/6 -> BusCreator/6  "PTC_Cfg Gearbox11 iFGear2"
  Demux/5 -> BusCreator/5  "PTC_Cfg Gearbox11 iFGear1"
  Demux/4 -> BusCreator/4  "PTC_Cfg Gearbox11 iFGear0"
  Demux/3 -> BusCreator/3  "PTC_Cfg Gearbox11 nFGears"
  Demux/2 -> BusCreator/2  "PTC_Cfg Gearbox11 ClKind"
  Demux/1 -> BusCreator/1  "PTC_Cfg Gearbox11 GBKind"
  BusCreator/1 -> Out/1
  In/1 -> Demux/1

== system generic_src/CarMaker/IPG Vehicle/PowerTrain/PTControl Example/PTControl_In/CreateBus PTC_Cfg Gearbox2 ==
  In : Inport
  BusCreator : BusCreator  Inputs=38
  Demux : Demux  Outputs=38
      settings: DisplayOption=none
  Out : Outport  VectorParamsAs1DForOutWhenUnconnected=off
  wires:
  Demux/38 -> BusCreator/38  "PTC_Cfg Gearbox2 iBGear16"
  Demux/37 -> BusCreator/37  "PTC_Cfg Gearbox2 iBGear15"
  Demux/36 -> BusCreator/36  "PTC_Cfg Gearbox2 iBGear14"
  Demux/35 -> BusCreator/35  "PTC_Cfg Gearbox2 iBGear13"
  Demux/34 -> BusCreator/34  "PTC_Cfg Gearbox2 iBGear12"
  Demux/33 -> BusCreator/33  "PTC_Cfg Gearbox2 iBGear11"
  Demux/32 -> BusCreator/32  "PTC_Cfg Gearbox2 iBGear10"
  Demux/31 -> BusCreator/31  "PTC_Cfg Gearbox2 iBGear9"
  Demux/30 -> BusCreator/30  "PTC_Cfg Gearbox2 iBGear8"
  Demux/29 -> BusCreator/29  "PTC_Cfg Gearbox2 iBGear7"
  Demux/28 -> BusCreator/28  "PTC_Cfg Gearbox2 iBGear6"
  Demux/27 -> BusCreator/27  "PTC_Cfg Gearbox2 iBGear5"
  Demux/26 -> BusCreator/26  "PTC_Cfg Gearbox2 iBGear4"
  Demux/25 -> BusCreator/25  "PTC_Cfg Gearbox2 iBGear3"
  Demux/24 -> BusCreator/24  "PTC_Cfg Gearbox2 iBGear2"
  Demux/23 -> BusCreator/23  "PTC_Cfg Gearbox2 iBGear1"
  Demux/22 -> BusCreator/22  "PTC_Cfg Gearbox2 iBGear0"
  Demux/21 -> BusCreator/21  "PTC_Cfg Gearbox2 nBGears"
  Demux/20 -> BusCreator/20  "PTC_Cfg Gearbox2 iFGear16"
  Demux/19 -> BusCreator/19  "PTC_Cfg Gearbox2 iFGear15"
  Demux/18 -> BusCreator/18  "PTC_Cfg Gearbox2 iFGear14"
  Demux/17 -> BusCreator/17  "PTC_Cfg Gearbox2 iFGear13"
  Demux/16 -> BusCreator/16  "PTC_Cfg Gearbox2 iFGear12"
  Demux/15 -> BusCreator/15  "PTC_Cfg Gearbox2 iFGear11"
  Demux/14 -> BusCreator/14  "PTC_Cfg Gearbox2 iFGear10"
  Demux/13 -> BusCreator/13  "PTC_Cfg Gearbox2 iFGear9"
  Demux/12 -> BusCreator/12  "PTC_Cfg Gearbox2 iFGear8"
  Demux/11 -> BusCreator/11  "PTC_Cfg Gearbox2 iFGear7"
  Demux/10 -> BusCreator/10  "PTC_Cfg Gearbox2 iFGear6"
  Demux/9 -> BusCreator/9  "PTC_Cfg Gearbox2 iFGear5"
  Demux/8 -> BusCreator/8  "PTC_Cfg Gearbox2 iFGear4"
  Demux/7 -> BusCreator/7  "PTC_Cfg Gearbox2 iFGear3"
  Demux/6 -> BusCreator/6  "PTC_Cfg Gearbox2 iFGear2"
  Demux/5 -> BusCreator/5  "PTC_Cfg Gearbox2 iFGear1"
  Demux/4 -> BusCreator/4  "PTC_Cfg Gearbox2 iFGear0"
  Demux/3 -> BusCreator/3  "PTC_Cfg Gearbox2 nFGears"
  Demux/2 -> BusCreator/2  "PTC_Cfg Gearbox2 ClKind"
  Demux/1 -> BusCreator/1  "PTC_Cfg Gearbox2 GBKind"
  BusCreator/1 -> Out/1
  In/1 -> Demux/1

== system generic_src/CarMaker/IPG Vehicle/PowerTrain/PTControl Example/PTControl_In/CreateBus PTC_Cfg Gearbox3 ==
  In : Inport
  BusCreator : BusCreator  Inputs=38
  Demux : Demux  Outputs=38
      settings: DisplayOption=none
  Out : Outport  VectorParamsAs1DForOutWhenUnconnected=off
  wires:
  Demux/38 -> BusCreator/38  "PTC_Cfg Gearbox3 iBGear16"
  Demux/37 -> BusCreator/37  "PTC_Cfg Gearbox3 iBGear15"
  Demux/36 -> BusCreator/36  "PTC_Cfg Gearbox3 iBGear14"
  Demux/35 -> BusCreator/35  "PTC_Cfg Gearbox3 iBGear13"
  Demux/34 -> BusCreator/34  "PTC_Cfg Gearbox3 iBGear12"
  Demux/33 -> BusCreator/33  "PTC_Cfg Gearbox3 iBGear11"
  Demux/32 -> BusCreator/32  "PTC_Cfg Gearbox3 iBGear10"
  Demux/31 -> BusCreator/31  "PTC_Cfg Gearbox3 iBGear9"
  Demux/30 -> BusCreator/30  "PTC_Cfg Gearbox3 iBGear8"
  Demux/29 -> BusCreator/29  "PTC_Cfg Gearbox3 iBGear7"
  Demux/28 -> BusCreator/28  "PTC_Cfg Gearbox3 iBGear6"
  Demux/27 -> BusCreator/27  "PTC_Cfg Gearbox3 iBGear5"
  Demux/26 -> BusCreator/26  "PTC_Cfg Gearbox3 iBGear4"
  Demux/25 -> BusCreator/25  "PTC_Cfg Gearbox3 iBGear3"
  Demux/24 -> BusCreator/24  "PTC_Cfg Gearbox3 iBGear2"
  Demux/23 -> BusCreator/23  "PTC_Cfg Gearbox3 iBGear1"
  Demux/22 -> BusCreator/22  "PTC_Cfg Gearbox3 iBGear0"
  Demux/21 -> BusCreator/21  "PTC_Cfg Gearbox3 nBGears"
  Demux/20 -> BusCreator/20  "PTC_Cfg Gearbox3 iFGear16"
  Demux/19 -> BusCreator/19  "PTC_Cfg Gearbox3 iFGear15"
  Demux/18 -> BusCreator/18  "PTC_Cfg Gearbox3 iFGear14"
  Demux/17 -> BusCreator/17  "PTC_Cfg Gearbox3 iFGear13"
  Demux/16 -> BusCreator/16  "PTC_Cfg Gearbox3 iFGear12"
  Demux/15 -> BusCreator/15  "PTC_Cfg Gearbox3 iFGear11"
  Demux/14 -> BusCreator/14  "PTC_Cfg Gearbox3 iFGear10"
  Demux/13 -> BusCreator/13  "PTC_Cfg Gearbox3 iFGear9"
  Demux/12 -> BusCreator/12  "PTC_Cfg Gearbox3 iFGear8"
  Demux/11 -> BusCreator/11  "PTC_Cfg Gearbox3 iFGear7"
  Demux/10 -> BusCreator/10  "PTC_Cfg Gearbox3 iFGear6"
  Demux/9 -> BusCreator/9  "PTC_Cfg Gearbox3 iFGear5"
  Demux/8 -> BusCreator/8  "PTC_Cfg Gearbox3 iFGear4"
  Demux/7 -> BusCreator/7  "PTC_Cfg Gearbox3 iFGear3"
  Demux/6 -> BusCreator/6  "PTC_Cfg Gearbox3 iFGear2"
  Demux/5 -> BusCreator/5  "PTC_Cfg Gearbox3 iFGear1"
  Demux/4 -> BusCreator/4  "PTC_Cfg Gearbox3 iFGear0"
  Demux/3 -> BusCreator/3  "PTC_Cfg Gearbox3 nFGears"
  Demux/2 -> BusCreator/2  "PTC_Cfg Gearbox3 ClKind"
  Demux/1 -> BusCreator/1  "PTC_Cfg Gearbox3 GBKind"
  BusCreator/1 -> Out/1
  In/1 -> Demux/1

== system generic_src/CarMaker/IPG Vehicle/PowerTrain/PTControl Example/PTControl_In/CreateBus PTC_Cfg Gearbox4 ==
  In : Inport
  BusCreator : BusCreator  Inputs=38
  Demux : Demux  Outputs=38
      settings: DisplayOption=none
  Out : Outport  VectorParamsAs1DForOutWhenUnconnected=off
  wires:
  Demux/38 -> BusCreator/38  "PTC_Cfg Gearbox4 iBGear16"
  Demux/37 -> BusCreator/37  "PTC_Cfg Gearbox4 iBGear15"
  Demux/36 -> BusCreator/36  "PTC_Cfg Gearbox4 iBGear14"
  Demux/35 -> BusCreator/35  "PTC_Cfg Gearbox4 iBGear13"
  Demux/34 -> BusCreator/34  "PTC_Cfg Gearbox4 iBGear12"
  Demux/33 -> BusCreator/33  "PTC_Cfg Gearbox4 iBGear11"
  Demux/32 -> BusCreator/32  "PTC_Cfg Gearbox4 iBGear10"
  Demux/31 -> BusCreator/31  "PTC_Cfg Gearbox4 iBGear9"
  Demux/30 -> BusCreator/30  "PTC_Cfg Gearbox4 iBGear8"
  Demux/29 -> BusCreator/29  "PTC_Cfg Gearbox4 iBGear7"
  Demux/28 -> BusCreator/28  "PTC_Cfg Gearbox4 iBGear6"
  Demux/27 -> BusCreator/27  "PTC_Cfg Gearbox4 iBGear5"
  Demux/26 -> BusCreator/26  "PTC_Cfg Gearbox4 iBGear4"
  Demux/25 -> BusCreator/25  "PTC_Cfg Gearbox4 iBGear3"
  Demux/24 -> BusCreator/24  "PTC_Cfg Gearbox4 iBGear2"
  Demux/23 -> BusCreator/23  "PTC_Cfg Gearbox4 iBGear1"
  Demux/22 -> BusCreator/22  "PTC_Cfg Gearbox4 iBGear0"
  Demux/21 -> BusCreator/21  "PTC_Cfg Gearbox4 nBGears"
  Demux/20 -> BusCreator/20  "PTC_Cfg Gearbox4 iFGear16"
  Demux/19 -> BusCreator/19  "PTC_Cfg Gearbox4 iFGear15"
  Demux/18 -> BusCreator/18  "PTC_Cfg Gearbox4 iFGear14"
  Demux/17 -> BusCreator/17  "PTC_Cfg Gearbox4 iFGear13"
  Demux/16 -> BusCreator/16  "PTC_Cfg Gearbox4 iFGear12"
  Demux/15 -> BusCreator/15  "PTC_Cfg Gearbox4 iFGear11"
  Demux/14 -> BusCreator/14  "PTC_Cfg Gearbox4 iFGear10"
  Demux/13 -> BusCreator/13  "PTC_Cfg Gearbox4 iFGear9"
  Demux/12 -> BusCreator/12  "PTC_Cfg Gearbox4 iFGear8"
  Demux/11 -> BusCreator/11  "PTC_Cfg Gearbox4 iFGear7"
  Demux/10 -> BusCreator/10  "PTC_Cfg Gearbox4 iFGear6"
  Demux/9 -> BusCreator/9  "PTC_Cfg Gearbox4 iFGear5"
  Demux/8 -> BusCreator/8  "PTC_Cfg Gearbox4 iFGear4"
  Demux/7 -> BusCreator/7  "PTC_Cfg Gearbox4 iFGear3"
  Demux/6 -> BusCreator/6  "PTC_Cfg Gearbox4 iFGear2"
  Demux/5 -> BusCreator/5  "PTC_Cfg Gearbox4 iFGear1"
  Demux/4 -> BusCreator/4  "PTC_Cfg Gearbox4 iFGear0"
  Demux/3 -> BusCreator/3  "PTC_Cfg Gearbox4 nFGears"
  Demux/2 -> BusCreator/2  "PTC_Cfg Gearbox4 ClKind"
  Demux/1 -> BusCreator/1  "PTC_Cfg Gearbox4 GBKind"
  BusCreator/1 -> Out/1
  In/1 -> Demux/1

== system generic_src/CarMaker/IPG Vehicle/PowerTrain/PTControl Example/PTControl_In/CreateBus PTC_Cfg Gearbox5 ==
  In : Inport
  BusCreator : BusCreator  Inputs=38
  Demux : Demux  Outputs=38
      settings: DisplayOption=none
  Out : Outport  VectorParamsAs1DForOutWhenUnconnected=off
  wires:
  Demux/38 -> BusCreator/38  "PTC_Cfg Gearbox5 iBGear16"
  Demux/37 -> BusCreator/37  "PTC_Cfg Gearbox5 iBGear15"
  Demux/36 -> BusCreator/36  "PTC_Cfg Gearbox5 iBGear14"
  Demux/35 -> BusCreator/35  "PTC_Cfg Gearbox5 iBGear13"
  Demux/34 -> BusCreator/34  "PTC_Cfg Gearbox5 iBGear12"
  Demux/33 -> BusCreator/33  "PTC_Cfg Gearbox5 iBGear11"
  Demux/32 -> BusCreator/32  "PTC_Cfg Gearbox5 iBGear10"
  Demux/31 -> BusCreator/31  "PTC_Cfg Gearbox5 iBGear9"
  Demux/30 -> BusCreator/30  "PTC_Cfg Gearbox5 iBGear8"
  Demux/29 -> BusCreator/29  "PTC_Cfg Gearbox5 iBGear7"
  Demux/28 -> BusCreator/28  "PTC_Cfg Gearbox5 iBGear6"
  Demux/27 -> BusCreator/27  "PTC_Cfg Gearbox5 iBGear5"
  Demux/26 -> BusCreator/26  "PTC_Cfg Gearbox5 iBGear4"
  Demux/25 -> BusCreator/25  "PTC_Cfg Gearbox5 iBGear3"
  Demux/24 -> BusCreator/24  "PTC_Cfg Gearbox5 iBGear2"
  Demux/23 -> BusCreator/23  "PTC_Cfg Gearbox5 iBGear1"
  Demux/22 -> BusCreator/22  "PTC_Cfg Gearbox5 iBGear0"
  Demux/21 -> BusCreator/21  "PTC_Cfg Gearbox5 nBGears"
  Demux/20 -> BusCreator/20  "PTC_Cfg Gearbox5 iFGear16"
  Demux/19 -> BusCreator/19  "PTC_Cfg Gearbox5 iFGear15"
  Demux/18 -> BusCreator/18  "PTC_Cfg Gearbox5 iFGear14"
  Demux/17 -> BusCreator/17  "PTC_Cfg Gearbox5 iFGear13"
  Demux/16 -> BusCreator/16  "PTC_Cfg Gearbox5 iFGear12"
  Demux/15 -> BusCreator/15  "PTC_Cfg Gearbox5 iFGear11"
  Demux/14 -> BusCreator/14  "PTC_Cfg Gearbox5 iFGear10"
  Demux/13 -> BusCreator/13  "PTC_Cfg Gearbox5 iFGear9"
  Demux/12 -> BusCreator/12  "PTC_Cfg Gearbox5 iFGear8"
  Demux/11 -> BusCreator/11  "PTC_Cfg Gearbox5 iFGear7"
  Demux/10 -> BusCreator/10  "PTC_Cfg Gearbox5 iFGear6"
  Demux/9 -> BusCreator/9  "PTC_Cfg Gearbox5 iFGear5"
  Demux/8 -> BusCreator/8  "PTC_Cfg Gearbox5 iFGear4"
  Demux/7 -> BusCreator/7  "PTC_Cfg Gearbox5 iFGear3"
  Demux/6 -> BusCreator/6  "PTC_Cfg Gearbox5 iFGear2"
  Demux/5 -> BusCreator/5  "PTC_Cfg Gearbox5 iFGear1"
  Demux/4 -> BusCreator/4  "PTC_Cfg Gearbox5 iFGear0"
  Demux/3 -> BusCreator/3  "PTC_Cfg Gearbox5 nFGears"
  Demux/2 -> BusCreator/2  "PTC_Cfg Gearbox5 ClKind"
  Demux/1 -> BusCreator/1  "PTC_Cfg Gearbox5 GBKind"
  BusCreator/1 -> Out/1
  In/1 -> Demux/1

== system generic_src/CarMaker/IPG Vehicle/PowerTrain/PTControl Example/PTControl_In/CreateBus PTC_Cfg Gearbox6 ==
  In : Inport
  BusCreator : BusCreator  Inputs=38
  Demux : Demux  Outputs=38
      settings: DisplayOption=none
  Out : Outport  VectorParamsAs1DForOutWhenUnconnected=off
  wires:
  Demux/38 -> BusCreator/38  "PTC_Cfg Gearbox6 iBGear16"
  Demux/37 -> BusCreator/37  "PTC_Cfg Gearbox6 iBGear15"
  Demux/36 -> BusCreator/36  "PTC_Cfg Gearbox6 iBGear14"
  Demux/35 -> BusCreator/35  "PTC_Cfg Gearbox6 iBGear13"
  Demux/34 -> BusCreator/34  "PTC_Cfg Gearbox6 iBGear12"
  Demux/33 -> BusCreator/33  "PTC_Cfg Gearbox6 iBGear11"
  Demux/32 -> BusCreator/32  "PTC_Cfg Gearbox6 iBGear10"
  Demux/31 -> BusCreator/31  "PTC_Cfg Gearbox6 iBGear9"
  Demux/30 -> BusCreator/30  "PTC_Cfg Gearbox6 iBGear8"
  Demux/29 -> BusCreator/29  "PTC_Cfg Gearbox6 iBGear7"
  Demux/28 -> BusCreator/28  "PTC_Cfg Gearbox6 iBGear6"
  Demux/27 -> BusCreator/27  "PTC_Cfg Gearbox6 iBGear5"
  Demux/26 -> BusCreator/26  "PTC_Cfg Gearbox6 iBGear4"
  Demux/25 -> BusCreator/25  "PTC_Cfg Gearbox6 iBGear3"
  Demux/24 -> BusCreator/24  "PTC_Cfg Gearbox6 iBGear2"
  Demux/23 -> BusCreator/23  "PTC_Cfg Gearbox6 iBGear1"
  Demux/22 -> BusCreator/22  "PTC_Cfg Gearbox6 iBGear0"
  Demux/21 -> BusCreator/21  "PTC_Cfg Gearbox6 nBGears"
  Demux/20 -> BusCreator/20  "PTC_Cfg Gearbox6 iFGear16"
  Demux/19 -> BusCreator/19  "PTC_Cfg Gearbox6 iFGear15"
  Demux/18 -> BusCreator/18  "PTC_Cfg Gearbox6 iFGear14"
  Demux/17 -> BusCreator/17  "PTC_Cfg Gearbox6 iFGear13"
  Demux/16 -> BusCreator/16  "PTC_Cfg Gearbox6 iFGear12"
  Demux/15 -> BusCreator/15  "PTC_Cfg Gearbox6 iFGear11"
  Demux/14 -> BusCreator/14  "PTC_Cfg Gearbox6 iFGear10"
  Demux/13 -> BusCreator/13  "PTC_Cfg Gearbox6 iFGear9"
  Demux/12 -> BusCreator/12  "PTC_Cfg Gearbox6 iFGear8"
  Demux/11 -> BusCreator/11  "PTC_Cfg Gearbox6 iFGear7"
  Demux/10 -> BusCreator/10  "PTC_Cfg Gearbox6 iFGear6"
  Demux/9 -> BusCreator/9  "PTC_Cfg Gearbox6 iFGear5"
  Demux/8 -> BusCreator/8  "PTC_Cfg Gearbox6 iFGear4"
  Demux/7 -> BusCreator/7  "PTC_Cfg Gearbox6 iFGear3"
  Demux/6 -> BusCreator/6  "PTC_Cfg Gearbox6 iFGear2"
  Demux/5 -> BusCreator/5  "PTC_Cfg Gearbox6 iFGear1"
  Demux/4 -> BusCreator/4  "PTC_Cfg Gearbox6 iFGear0"
  Demux/3 -> BusCreator/3  "PTC_Cfg Gearbox6 nFGears"
  Demux/2 -> BusCreator/2  "PTC_Cfg Gearbox6 ClKind"
  Demux/1 -> BusCreator/1  "PTC_Cfg Gearbox6 GBKind"
  BusCreator/1 -> Out/1
  In/1 -> Demux/1

== system generic_src/CarMaker/IPG Vehicle/PowerTrain/PTControl Example/PTControl_In/CreateBus PTC_Cfg Gearbox7 ==
  In : Inport
  BusCreator : BusCreator  Inputs=38
  Demux : Demux  Outputs=38
      settings: DisplayOption=none
  Out : Outport  VectorParamsAs1DForOutWhenUnconnected=off
  wires:
  Demux/38 -> BusCreator/38  "PTC_Cfg Gearbox7 iBGear16"
  Demux/37 -> BusCreator/37  "PTC_Cfg Gearbox7 iBGear15"
  Demux/36 -> BusCreator/36  "PTC_Cfg Gearbox7 iBGear14"
  Demux/35 -> BusCreator/35  "PTC_Cfg Gearbox7 iBGear13"
  Demux/34 -> BusCreator/34  "PTC_Cfg Gearbox7 iBGear12"
  Demux/33 -> BusCreator/33  "PTC_Cfg Gearbox7 iBGear11"
  Demux/32 -> BusCreator/32  "PTC_Cfg Gearbox7 iBGear10"
  Demux/31 -> BusCreator/31  "PTC_Cfg Gearbox7 iBGear9"
  Demux/30 -> BusCreator/30  "PTC_Cfg Gearbox7 iBGear8"
  Demux/29 -> BusCreator/29  "PTC_Cfg Gearbox7 iBGear7"
  Demux/28 -> BusCreator/28  "PTC_Cfg Gearbox7 iBGear6"
  Demux/27 -> BusCreator/27  "PTC_Cfg Gearbox7 iBGear5"
  Demux/26 -> BusCreator/26  "PTC_Cfg Gearbox7 iBGear4"
  Demux/25 -> BusCreator/25  "PTC_Cfg Gearbox7 iBGear3"
  Demux/24 -> BusCreator/24  "PTC_Cfg Gearbox7 iBGear2"
  Demux/23 -> BusCreator/23  "PTC_Cfg Gearbox7 iBGear1"
  Demux/22 -> BusCreator/22  "PTC_Cfg Gearbox7 iBGear0"
  Demux/21 -> BusCreator/21  "PTC_Cfg Gearbox7 nBGears"
  Demux/20 -> BusCreator/20  "PTC_Cfg Gearbox7 iFGear16"
  Demux/19 -> BusCreator/19  "PTC_Cfg Gearbox7 iFGear15"
  Demux/18 -> BusCreator/18  "PTC_Cfg Gearbox7 iFGear14"
  Demux/17 -> BusCreator/17  "PTC_Cfg Gearbox7 iFGear13"
  Demux/16 -> BusCreator/16  "PTC_Cfg Gearbox7 iFGear12"
  Demux/15 -> BusCreator/15  "PTC_Cfg Gearbox7 iFGear11"
  Demux/14 -> BusCreator/14  "PTC_Cfg Gearbox7 iFGear10"
  Demux/13 -> BusCreator/13  "PTC_Cfg Gearbox7 iFGear9"
  Demux/12 -> BusCreator/12  "PTC_Cfg Gearbox7 iFGear8"
  Demux/11 -> BusCreator/11  "PTC_Cfg Gearbox7 iFGear7"
  Demux/10 -> BusCreator/10  "PTC_Cfg Gearbox7 iFGear6"
  Demux/9 -> BusCreator/9  "PTC_Cfg Gearbox7 iFGear5"
  Demux/8 -> BusCreator/8  "PTC_Cfg Gearbox7 iFGear4"
  Demux/7 -> BusCreator/7  "PTC_Cfg Gearbox7 iFGear3"
  Demux/6 -> BusCreator/6  "PTC_Cfg Gearbox7 iFGear2"
  Demux/5 -> BusCreator/5  "PTC_Cfg Gearbox7 iFGear1"
  Demux/4 -> BusCreator/4  "PTC_Cfg Gearbox7 iFGear0"
  Demux/3 -> BusCreator/3  "PTC_Cfg Gearbox7 nFGears"
  Demux/2 -> BusCreator/2  "PTC_Cfg Gearbox7 ClKind"
  Demux/1 -> BusCreator/1  "PTC_Cfg Gearbox7 GBKind"
  BusCreator/1 -> Out/1
  In/1 -> Demux/1
